simulink model "proxy_linux"  (R2017b)
settings: Solver=ode3  StartTime=0.0  StopTime=inf  FixedStep=0.01  RelTol=1e-3  EnableMultiTasking=on
model workspace (MAT data in the model file):
  SL_ROS_VariableLengthArrays_MaxSizes : struct (value not decoded)
undefined symbols (not defined in the file or in its folder): ampliFactor, ampliFactorDistal, ampliFactorMiddle, filt
libraries: robotlib x11, simulink_extras x11, simulink x8, etargetslib x4, dspnetwork x4
(part 3 of 6)

== matlab function proxy_linux/Generate SchunkCommands /Index Finger/New Version/Jacobian2 ==
  data: pose input; sensor input; measurements input; JTcomp output single; q_next output; q_pr input; J22_old input; J22_ol output
function [JTcomp, q_next, J22_ol] = fcn( pose, sensor, measurements, q_pr, J22_old)
%#codegen
% JTcomp_T = zeros(1,2);
%JTcomp = zeros(1,2);

lx = sensor(1);
qB = sensor(2);

qo1 =pose(1);
qo2 =pose(2);
qK = pose(3);
qD = pose(4);
qG = pose(5);
qN = pose(6);
c1 = pose(7);
c2 = pose(8);

%POSE ESTIMATION VALUE
LIIp = measurements(2);
LJJp = LIIp;
LLM = measurements(1);

%LIIp= measurements(1);
%LJJp = measurements(2);
%LLM = measurements(3);
%offset = measurements(4);
%xL = measurements(5);


% LIIp = 7;
% LJJp = LIIp;
% LLM = 50;
% offset = 3;
xL = 10;

f1 = LLM;
f5 = xL;
LBH = 37; 
LKB = 35;
LKH = LKB + LBH;
LCI = 16;
LGH =  86;
LHG =  LGH;
LDE = 40;
LAB =  18;   
LEF =  27;
LGF =  46;
LCD =  9;
LBC =  43;
oy  = 134.8;
ox  = 15; 
LEJ =  39;
off_fing = LIIp;  
lact = 117.77;
% LKN =  135.6320;
LNO = lact;
LDF = LDE + LEF;
LBD = LBC + LCD;


stepsize = 0.01;

%%NEWEST (Jacobian_StiffnessRenderingOptimization_Sim.mdl)
q_dif = (sensor - q_pr) / stepsize;
q_dif1 = q_dif(1);
q_dif2 = q_dif(2);


J11 = -(cos(qo1)*(LKB*cos(qK)+LBC*cos(qB-qK)-LCI*sin(qB-qK))-sin(qo1)*(LKB*sin(qK)-LBC*sin(qB-qK)-LCI*cos(qB-qK)))*((LDE+LEF)*sin(qo2)*cos(qB-qD-qG)*(LKB*sin(qK)-LBC*sin(qB-qK)-LCI*cos(qB-qK))+(LDE+LEF)*sin(qN)^2*cos(qB-qD-qG)*(cos(qo1)*sin(qo1+qo2)*(LKB*sin(qK)-LBC*sin(qB-qK))-LCI*cos(qo1)*sin(qo1+qo2)*cos(qB-qK)-sin(qo2)*(LKB*sin(qK)-LBC*sin(qB-qK)-LCI*cos(qB-qK))-sin(qo1)*cos(qo1+qo2)*(LKB*sin(qK)-LBC*sin(qB-qK)-LCI*cos(qB-qK)))-cos(qo1)*((LDE+LEF)*cos(qB-qD-qG)*(cos(qo1+qo2)*(LCD*cos(qB-qK)+LCI*sin(qB-qK)+LDE*cos(qB-qD-qK)-LEJ*sin(qB-qD-qK))-sin(qo1+qo2)*(LCI*cos(qB-qK)-LCD*sin(qB-qK)-LDE*sin(qB-qD-qK)-LEJ*cos(qB-qD-qK)))+(sin(qo1+qo2)*(LDE*sin(qB-qD-qK)+LEJ*cos(qB-qD-qK))+cos(qo1+qo2)*(LDE*cos(qB-qD-qK)-LEJ*sin(qB-qD-qK)))*(cos(qG-qK)*(LBH*cos(qK)+LHG*sin(qK)-LBC*cos(qB-qK)-LCD*cos(qB-qK)-LDE*cos(qB-qD-qK)-LEF*cos(qB-qD-qK))+sin(qG-qK)*(LHG*cos(qK)-LBH*sin(qK)-LBC*sin(qB-qK)-LCD*sin(qB-qK)-LDE*sin(qB-qD-qK)-LEF*sin(qB-qD-qK)))))/(cos(qN)*(LKB*sin(qK)+LAB*sin(qB-qK)-tan(qN)*(LKB*cos(qK)-LAB*cos(qB-qK)))*((LDE+LEF)*sin(qo1)*sin(qo2)*cos(qB-qD-qG)*(LIIp*cos(qo1)-c1*sin(qo1))*(LKB*sin(qK)-LBC*sin(qB-qK)-LCI*cos(qB-qK))-cos(qo1)*((LIIp*sin(qo1)+c1*cos(qo1))*((LDE+LEF)*sin(qo2)*cos(qB-qD-qG)*(LKB*sin(qK)-LBC*sin(qB-qK)-LCI*cos(qB-qK))-cos(qo1)*((LDE+LEF)*cos(qB-qD-qG)*(cos(qo1+qo2)*(LCD*cos(qB-qK)+LCI*sin(qB-qK)+LDE*cos(qB-qD-qK)-LEJ*sin(qB-qD-qK))-sin(qo1+qo2)*(LCI*cos(qB-qK)-LCD*sin(qB-qK)-LDE*sin(qB-qD-qK)-LEJ*cos(qB-qD-qK)))+(sin(qo1+qo2)*(LDE*sin(qB-qD-qK)+LEJ*cos(qB-qD-qK))+cos(qo1+qo2)*(LDE*cos(qB-qD-qK)-LEJ*sin(qB-qD-qK)))*(cos(qG-qK)*(LBH*cos(qK)+LHG*sin(qK)-LBC*cos(qB-qK)-LCD*cos(qB-qK)-LDE*cos(qB-qD-qK)-LEF*cos(qB-qD-qK))+sin(qG-qK)*(LHG*cos(qK)-LBH*sin(qK)-LBC*sin(qB-qK)-LCD*sin(qB-qK)-LDE*sin(qB-qD-qK)-LEF*sin(qB-qD-qK)))))-sin(qo1)*(LIIp*cos(qo1)-c1*sin(qo1))*((LDE+LEF)*sin(qo1+qo2)*cos(qB-qD-qG)*(LCI*cos(qB-qK)-LCD*sin(qB-qK)-LDE*sin(qB-qD-qK)-LEJ*cos(qB-qD-qK))-sin(qo1+qo2)*(LDE*sin(qB-qD-qK)+LEJ*cos(qB-qD-qK))*(cos(qG-qK)*(LBH*cos(qK)+LHG*sin(qK)-LBC*cos(qB-qK)-LCD*cos(qB-qK)-LDE*cos(qB-qD-qK)-LEF*cos(qB-qD-qK))+sin(qG-qK)*(LHG*cos(qK)-LBH*sin(qK)-LBC*sin(qB-qK)-LCD*sin(qB-qK)-LDE*sin(qB-qD-qK)-LEF*sin(qB-qD-qK)))-cos(qo1+qo2)*((LDE+LEF)*cos(qG-qK)*cos(qB-qD-qK)*(LCD*cos(qB-qK)+LCI*sin(qB-qK)+LDE*cos(qB-qD-qK)-LEJ*sin(qB-qD-qK))+cos(qG-qK)*(LDE*cos(qB-qD-qK)-LEJ*sin(qB-qD-qK))*(LBH*cos(qK)+LHG*sin(qK)-LBC*cos(qB-qK)-LCD*cos(qB-qK)-LDE*cos(qB-qD-qK)-LEF*cos(qB-qD-qK))+sin(qG-qK)*((LDE+LEF)*sin(qB-qD-qK)*(LCD*cos(qB-qK)+LCI*sin(qB-qK)+LDE*cos(qB-qD-qK)-LEJ*sin(qB-qD-qK))+(LDE*cos(qB-qD-qK)-LEJ*sin(qB-qD-qK))*(LHG*cos(qK)-LBH*sin(qK)-LBC*sin(qB-qK)-LCD*sin(qB-qK)-LDE*sin(qB-qD-qK)-LEF*sin(qB-qD-qK))))))));
J12 = cos(qo1)*((LDE+LEF)*sin(qo1+qo2)*cos(qB-qD-qG)*(LCI*cos(qB-qK)-LCD*sin(qB-qK)-LDE*sin(qB-qD-qK)-LEJ*cos(qB-qD-qK))*(cos(qo1)*(LKB*cos(qK)+LBC*cos(qB-qK)-LCI*sin(qB-qK))-sin(qo1)*(LKB*sin(qK)-LBC*sin(qB-qK)-LCI*cos(qB-qK)))+sin(qG-qK)*(LBC*sin(qB-qK)+LCD*sin(qB-qK)+LDE*sin(qB-qD-qK)+LEF*sin(qB-qD-qK))*(sin(qo1+qo2)*(LDE*sin(qB-qD-qK)+LEJ*cos(qB-qD-qK))+cos(qo1+qo2)*(LDE*cos(qB-qD-qK)-LEJ*sin(qB-qD-qK)))*(cos(qo1)*(LKB*cos(qK)+LBC*cos(qB-qK)-LCI*sin(qB-qK))-sin(qo1)*(LKB*sin(qK)-LBC*sin(qB-qK)-LCI*cos(qB-qK)))+cos(qG-qK)*(LBC*cos(qB-qK)+LCD*cos(qB-qK)+LDE*cos(qB-qD-qK)+LEF*cos(qB-qD-qK))*(sin(qo1+qo2)*(LDE*sin(qB-qD-qK)+LEJ*cos(qB-qD-qK))+cos(qo1+qo2)*(LDE*cos(qB-qD-qK)-LEJ*sin(qB-qD-qK)))*(cos(qo1)*(LKB*cos(qK)+LBC*cos(qB-qK)-LCI*sin(qB-qK))-sin(qo1)*(LKB*sin(qK)-LBC*sin(qB-qK)-LCI*cos(qB-qK)))-(LDE+LEF)*cos(qo1+qo2)*cos(qB-qD-qG)*(LCD*cos(qB-qK)+LCI*sin(qB-qK)+LDE*cos(qB-qD-qK)-LEJ*sin(qB-qD-qK))*(cos(qo1)*(LKB*cos(qK)+LBC*cos(qB-qK)-LCI*sin(qB-qK))-sin(qo1)*(LKB*sin(qK)-LBC*sin(qB-qK)-LCI*cos(qB-qK)))-(LBC*cos(qB-qK)-LCI*sin(qB-qK))*((LDE+LEF)*sin(qo2)*cos(qB-qD-qG)*(LKB*sin(qK)-LBC*sin(qB-qK)-LCI*cos(qB-qK))-cos(qo1)*((LDE+LEF)*cos(qB-qD-qG)*(cos(qo1+qo2)*(LCD*cos(qB-qK)+LCI*sin(qB-qK)+LDE*cos(qB-qD-qK)-LEJ*sin(qB-qD-qK))-sin(qo1+qo2)*(LCI*cos(qB-qK)-LCD*sin(qB-qK)-LDE*sin(qB-qD-qK)-LEJ*cos(qB-qD-qK)))+(sin(qo1+qo2)*(LDE*sin(qB-qD-qK)+LEJ*cos(qB-qD-qK))+cos(qo1+qo2)*(LDE*cos(qB-qD-qK)-LEJ*sin(qB-qD-qK)))*(cos(qG-qK)*(LBH*cos(qK)+LHG*sin(qK)-LBC*cos(qB-qK)-LCD*cos(qB-qK)-LDE*cos(qB-qD-qK)-LEF*cos(qB-qD-qK))+sin(qG-qK)*(LHG*cos(qK)-LBH*sin(qK)-LBC*sin(qB-qK)-LCD*sin(qB-qK)-LDE*sin(qB-qD-qK)-LEF*sin(qB-qD-qK)))))-(LBC*sin(qB-qK)+LCI*cos(qB-qK))*((LDE+LEF)*sin(qo2)*cos(qB-qD-qG)*(LKB*cos(qK)+LBC*cos(qB-qK)-LCI*sin(qB-qK))+sin(qo1)*((LDE+LEF)*sin(qo1+qo2)*cos(qB-qD-qG)*(LCI*cos(qB-qK)-LCD*sin(qB-qK)-LDE*sin(qB-qD-qK)-LEJ*cos(qB-qD-qK))-sin(qo1+qo2)*(LDE*sin(qB-qD-qK)+LEJ*cos(qB-qD-qK))*(cos(qG-qK)*(LBH*cos(qK)+LHG*sin(qK)-LBC*cos(qB-qK)-LCD*cos(qB-qK)-LDE*cos(qB-qD-qK)-LEF*cos(qB-qD-qK))+sin(qG-qK)*(LHG*cos(qK)-LBH*sin(qK)-LBC*sin(qB-qK)-LCD*sin(qB-qK)-LDE*sin(qB-qD-qK)-LEF*sin(qB-qD-qK)))-cos(qo1+qo2)*((LDE+LEF)*cos(qG-qK)*cos(qB-qD-qK)*(LCD*cos(qB-qK)+LCI*sin(qB-qK)+LDE*cos(qB-qD-qK)-LEJ*sin(qB-qD-qK))+cos(qG-qK)*(LDE*cos(qB-qD-qK)-LEJ*sin(qB-qD-qK))*(LBH*cos(qK)+LHG*sin(qK)-LBC*cos(qB-qK)-LCD*cos(qB-qK)-LDE*cos(qB-qD-qK)-LEF*cos(qB-qD-qK))+sin(qG-qK)*((LDE+LEF)*sin(qB-qD-qK)*(LCD*cos(qB-qK)+LCI*sin(qB-qK)+LDE*cos(qB-qD-qK)-LEJ*sin(qB-qD-qK))+(LDE*cos(qB-qD-qK)-LEJ*sin(qB-qD-qK))*(LHG*cos(qK)-LBH*sin(qK)-LBC*sin(qB-qK)-LCD*sin(qB-qK)-LDE*sin(qB-qD-qK)-LEF*sin(qB-qD-qK)))))))/((LDE+LEF)*sin(qo1)*sin(qo2)*cos(qB-qD-qG)*(LIIp*cos(qo1)-c1*sin(qo1))*(LKB*sin(qK)-LBC*sin(qB-qK)-LCI*cos(qB-qK))-cos(qo1)*((LIIp*sin(qo1)+c1*cos(qo1))*((LDE+LEF)*sin(qo2)*cos(qB-qD-qG)*(LKB*sin(qK)-LBC*sin(qB-qK)-LCI*cos(qB-qK))-cos(qo1)*((LDE+LEF)*cos(qB-qD-qG)*(cos(qo1+qo2)*(LCD*cos(qB-qK)+LCI*sin(qB-qK)+LDE*cos(qB-qD-qK)-LEJ*sin(qB-qD-qK))-sin(qo1+qo2)*(LCI*cos(qB-qK)-LCD*sin(qB-qK)-LDE*sin(qB-qD-qK)-LEJ*cos(qB-qD-qK)))+(sin(qo1+qo2)*(LDE*sin(qB-qD-qK)+LEJ*cos(qB-qD-qK))+cos(qo1+qo2)*(LDE*cos(qB-qD-qK)-LEJ*sin(qB-qD-qK)))*(cos(qG-qK)*(LBH*cos(qK)+LHG*sin(qK)-LBC*cos(qB-qK)-LCD*cos(qB-qK)-LDE*cos(qB-qD-qK)-LEF*cos(qB-qD-qK))+sin(qG-qK)*(LHG*cos(qK)-LBH*sin(qK)-LBC*sin(qB-qK)-LCD*sin(qB-qK)-LDE*sin(qB-qD-qK)-LEF*sin(qB-qD-qK)))))-sin(qo1)*(LIIp*cos(qo1)-c1*sin(qo1))*((LDE+LEF)*sin(qo1+qo2)*cos(qB-qD-qG)*(LCI*cos(qB-qK)-LCD*sin(qB-qK)-LDE*sin(qB-qD-qK)-LEJ*cos(qB-qD-qK))-sin(qo1+qo2)*(LDE*sin(qB-qD-qK)+LEJ*cos(qB-qD-qK))*(cos(qG-qK)*(LBH*cos(qK)+LHG*sin(qK)-LBC*cos(qB-qK)-LCD*cos(qB-qK)-LDE*cos(qB-qD-qK)-LEF*cos(qB-qD-qK))+sin(qG-qK)*(LHG*cos(qK)-LBH*sin(qK)-LBC*sin(qB-qK)-LCD*sin(qB-qK)-LDE*sin(qB-qD-qK)-LEF*sin(qB-qD-qK)))-cos(qo1+qo2)*((LDE+LEF)*cos(qG-qK)*cos(qB-qD-qK)*(LCD*cos(qB-qK)+LCI*sin(qB-qK)+LDE*cos(qB-qD-qK)-LEJ*sin(qB-qD-qK))+cos(qG-qK)*(LDE*cos(qB-qD-qK)-LEJ*sin(qB-qD-qK))*(LBH*cos(qK)+LHG*sin(qK)-LBC*cos(qB-qK)-LCD*cos(qB-qK)-LDE*cos(qB-qD-qK)-LEF*cos(qB-qD-qK))+sin(qG-qK)*((LDE+LEF)*sin(qB-qD-qK)*(LCD*cos(qB-qK)+LCI*sin(qB-qK)+LDE*cos(qB-qD-qK)-LEJ*sin(qB-qD-qK))+(LDE*cos(qB-qD-qK)-LEJ*sin(qB-qD-qK))*(LHG*cos(qK)-LBH*sin(qK)-LBC*sin(qB-qK)-LCD*sin(qB-qK)-LDE*sin(qB-qD-qK)-LEF*sin(qB-qD-qK))))))) - (cos(qo1)*(LKB*cos(qK)+LBC*cos(qB-qK)-LCI*sin(qB-qK))-sin(qo1)*(LKB*sin(qK)-LBC*sin(qB-qK)-LCI*cos(qB-qK)))*((LDE+LEF)*cos(qo1)*sin(qo1+qo2)*cos(qB-qD-qG)*(LKB*sin(qK)+LAB*sin(qB-qK)-tan(qN)*(LKB*cos(qK)-LAB*cos(qB-qK)))*(LCI*cos(qB-qK)-LCD*sin(qB-qK)-LDE*sin(qB-qD-qK)-LEJ*cos(qB-qD-qK))+cos(qo1)*sin(qG-qK)*(LKB*sin(qK)+LAB*sin(qB-qK)-tan(qN)*(LKB*cos(qK)-LAB*cos(qB-qK)))*(LBC*sin(qB-qK)+LCD*sin(qB-qK)+LDE*sin(qB-qD-qK)+LEF*sin(qB-qD-qK))*(sin(qo1+qo2)*(LDE*sin(qB-qD-qK)+LEJ*cos(qB-qD-qK))+cos(qo1+qo2)*(LDE*cos(qB-qD-qK)-LEJ*sin(qB-qD-qK)))+cos(qo1)*cos(qG-qK)*(LKB*sin(qK)+LAB*sin(qB-qK)-tan(qN)*(LKB*cos(qK)-LAB*cos(qB-qK)))*(LBC*cos(qB-qK)+LCD*cos(qB-qK)+LDE*cos(qB-qD-qK)+LEF*cos(qB-qD-qK))*(sin(qo1+qo2)*(LDE*sin(qB-qD-qK)+LEJ*cos(qB-qD-qK))+cos(qo1+qo2)*(LDE*cos(qB-qD-qK)-LEJ*sin(qB-qD-qK)))-(LDE+LEF)*sin(qo2)*cos(qB-qD-qG)*(LBC*sin(qB-qK)+LCI*cos(qB-qK))*(LKB*sin(qK)+LAB*sin(qB-qK)-tan(qN)*(LKB*cos(qK)-LAB*cos(qB-qK)))-(LDE+LEF)*cos(qo1)*cos(qo1+qo2)*cos(qB-qD-qG)*(LKB*sin(qK)+LAB*sin(qB-qK)-tan(qN)*(LKB*cos(qK)-LAB*cos(qB-qK)))*(LCD*cos(qB-qK)+LCI*sin(qB-qK)+LDE*cos(qB-qD-qK)-LEJ*sin(qB-qD-qK))-LAB*sin(qB-qK)*((LDE+LEF)*sin(qo2)*cos(qB-qD-qG)*(LKB*sin(qK)-LBC*sin(qB-qK)-LCI*cos(qB-qK))-cos(qo1)*((LDE+LEF)*cos(qB-qD-qG)*(cos(qo1+qo2)*(LCD*cos(qB-qK)+LCI*sin(qB-qK)+LDE*cos(qB-qD-qK)-LEJ*sin(qB-qD-qK))-sin(qo1+qo2)*(LCI*cos(qB-qK)-LCD*sin(qB-qK)-LDE*sin(qB-qD-qK)-LEJ*cos(qB-qD-qK)))+(sin(qo1+qo2)*(LDE*sin(qB-qD-qK)+LEJ*cos(qB-qD-qK))+cos(qo1+qo2)*(LDE*cos(qB-qD-qK)-LEJ*sin(qB-qD-qK)))*(cos(qG-qK)*(LBH*cos(qK)+LHG*sin(qK)-LBC*cos(qB-qK)-LCD*cos(qB-qK)-LDE*cos(qB-qD-qK)-LEF*cos(qB-qD-qK))+sin(qG-qK)*(LHG*cos(qK)-LBH*sin(qK)-LBC*sin(qB-qK)-LCD*sin(qB-qK)-LDE*sin(qB-qD-qK)-LEF*sin(qB-qD-qK)))))-LAB*tan(qN)*cos(qB-qK)*((LDE+LEF)*cos(qo1)*sin(qo1+qo2)*cos(qB-qD-qG)*(LKB*sin(qK)-LBC*sin(qB-qK)-LCD*sin(qB-qK)-LDE*sin(qB-qD-qK)-LEJ*cos(qB-qD-qK))-(LDE+LEF)*sin(qo1)*cos(qo1+qo2)*cos(qB-qD-qG)*(LKB*sin(qK)-LBC*sin(qB-qK)-LCI*cos(qB-qK))-cos(qo1)*sin(qo1+qo2)*(LDE*sin(qB-qD-qK)+LEJ*cos(qB-qD-qK))*(cos(qG-qK)*(LBH*cos(qK)+LHG*sin(qK)-LBC*cos(qB-qK)-LCD*cos(qB-qK)-LDE*cos(qB-qD-qK)-LEF*cos(qB-qD-qK))+sin(qG-qK)*(LHG*cos(qK)-LBH*sin(qK)-LBC*sin(qB-qK)-LCD*sin(qB-qK)-LDE*sin(qB-qD-qK)-LEF*sin(qB-qD-qK)))-cos(qo1)*cos(qo1+qo2)*((LDE+LEF)*cos(qG-qK)*cos(qB-qD-qK)*(LCD*cos(qB-qK)+LCI*sin(qB-qK)+LDE*cos(qB-qD-qK)-LEJ*sin(qB-qD-qK))+cos(qG-qK)*(LDE*cos(qB-qD-qK)-LEJ*sin(qB-qD-qK))*(LBH*cos(qK)+LHG*sin(qK)-LBC*cos(qB-qK)-LCD*cos(qB-qK)-LDE*cos(qB-qD-qK)-LEF*cos(qB-qD-qK))+sin(qG-qK)*((LDE+LEF)*sin(qB-qD-qK)*(LCD*cos(qB-qK)+LCI*sin(qB-qK)+LDE*cos(qB-qD-qK)-LEJ*sin(qB-qD-qK))+(LDE*cos(qB-qD-qK)-LEJ*sin(qB-qD-qK))*(LHG*cos(qK)-LBH*sin(qK)-LBC*sin(qB-qK)-LCD*sin(qB-qK)-LDE*sin(qB-qD-qK)-LEF*sin(qB-qD-qK))))))/((LKB*sin(qK)+LAB*sin(qB-qK)-tan(qN)*(LKB*cos(qK)-LAB*cos(qB-qK)))*((LDE+LEF)*sin(qo1)*sin(qo2)*cos(qB-qD-qG)*(LIIp*cos(qo1)-c1*sin(qo1))*(LKB*sin(qK)-LBC*sin(qB-qK)-LCI*cos(qB-qK))-cos(qo1)*((LIIp*sin(qo1)+c1*cos(qo1))*((LDE+LEF)*sin(qo2)*cos(qB-qD-qG)*(LKB*sin(qK)-LBC*sin(qB-qK)-LCI*cos(qB-qK))-cos(qo1)*((LDE+LEF)*cos(qB-qD-qG)*(cos(qo1+qo2)*(LCD*cos(qB-qK)+LCI*sin(qB-qK)+LDE*cos(qB-qD-qK)-LEJ*sin(qB-qD-qK))-sin(qo1+qo2)*(LCI*cos(qB-qK)-LCD*sin(qB-qK)-LDE*sin(qB-qD-qK)-LEJ*cos(qB-qD-qK)))+(sin(qo1+qo2)*(LDE*sin(qB-qD-qK)+LEJ*cos(qB-qD-qK))+cos(qo1+qo2)*(LDE*cos(qB-qD-qK)-LEJ*sin(qB-qD-qK)))*(cos(qG-qK)*(LBH*cos(qK)+LHG*sin(qK)-LBC*cos(qB-qK)-LCD*cos(qB-qK)-LDE*cos(qB-qD-qK)-LEF*cos(qB-qD-qK))+sin(qG-qK)*(LHG*cos(qK)-LBH*sin(qK)-LBC*sin(qB-qK)-LCD*sin(qB-qK)-LDE*sin(qB-qD-qK)-LEF*sin(qB-qD-qK)))))-sin(qo1)*(LIIp*cos(qo1)-c1*sin(qo1))*((LDE+LEF)*sin(qo1+qo2)*cos(qB-qD-qG)*(LCI*cos(qB-qK)-LCD*sin(qB-qK)-LDE*sin(qB-qD-qK)-LEJ*cos(qB-qD-qK))-sin(qo1+qo2)*(LDE*sin(qB-qD-qK)+LEJ*cos(qB-qD-qK))*(cos(qG-qK)*(LBH*cos(qK)+LHG*sin(qK)-LBC*cos(qB-qK)-LCD*cos(qB-qK)-LDE*cos(qB-qD-qK)-LEF*cos(qB-qD-qK))+sin(qG-qK)*(LHG*cos(qK)-LBH*sin(qK)-LBC*sin(qB-qK)-LCD*sin(qB-qK)-LDE*sin(qB-qD-qK)-LEF*sin(qB-qD-qK)))-cos(qo1+qo2)*((LDE+LEF)*cos(qG-qK)*cos(qB-qD-qK)*(LCD*cos(qB-qK)+LCI*sin(qB-qK)+LDE*cos(qB-qD-qK)-LEJ*sin(qB-qD-qK))+cos(qG-qK)*(LDE*cos(qB-qD-qK)-LEJ*sin(qB-qD-qK))*(LBH*cos(qK)+LHG*sin(qK)-LBC*cos(qB-qK)-LCD*cos(qB-qK)-LDE*cos(qB-qD-qK)-LEF*cos(qB-qD-qK))+sin(qG-qK)*((LDE+LEF)*sin(qB-qD-qK)*(LCD*cos(qB-qK)+LCI*sin(qB-qK)+LDE*cos(qB-qD-qK)-LEJ*sin(qB-qD-qK))+(LDE*cos(qB-qD-qK)-LEJ*sin(qB-qD-qK))*(LHG*cos(qK)-LBH*sin(qK)-LBC*sin(qB-qK)-LCD*sin(qB-qK)-LDE*sin(qB-qD-qK)-LEF*sin(qB-qD-qK))))))));
J21 = -(((LDE+LEF)*sin(qo2)*cos(qB-qD-qG)*(LKB*sin(qK)-LBC*sin(qB-qK)-LCI*cos(qB-qK))-cos(qo1)*((LDE+LEF)*cos(qB-qD-qG)*(cos(qo1+qo2)*(LCD*cos(qB-qK)+LCI*sin(qB-qK)+LDE*cos(qB-qD-qK)-LEJ*sin(qB-qD-qK))-sin(qo1+qo2)*(LCI*cos(qB-qK)-LCD*sin(qB-qK)-LDE*sin(qB-qD-qK)-LEJ*cos(qB-qD-qK)))+(sin(qo1+qo2)*(LDE*sin(qB-qD-qK)+LEJ*cos(qB-qD-qK))+cos(qo1+qo2)*(LDE*cos(qB-qD-qK)-LEJ*sin(qB-qD-qK)))*(cos(qG-qK)*(LBH*cos(qK)+LHG*sin(qK)-LBC*cos(qB-qK)-LCD*cos(qB-qK)-LDE*cos(qB-qD-qK)-LEF*cos(qB-qD-qK))+sin(qG-qK)*(LHG*cos(qK)-LBH*sin(qK)-LBC*sin(qB-qK)-LCD*sin(qB-qK)-LDE*sin(qB-qD-qK)-LEF*sin(qB-qD-qK)))))^2*(cos(qN)+sin(qN)^2*((LDE+LEF)*cos(qo1)*sin(qo1+qo2)*cos(qB-qD-qG)*(LKB*sin(qK)-LBC*sin(qB-qK)-LCD*sin(qB-qK)-LDE*sin(qB-qD-qK)-LEJ*cos(qB-qD-qK))-(LDE+LEF)*sin(qo1)*cos(qo1+qo2)*cos(qB-qD-qG)*(LKB*sin(qK)-LBC*sin(qB-qK)-LCI*cos(qB-qK))-cos(qo1)*sin(qo1+qo2)*(LDE*sin(qB-qD-qK)+LEJ*cos(qB-qD-qK))*(cos(qG-qK)*(LBH*cos(qK)+LHG*sin(qK)-LBC*cos(qB-qK)-LCD*cos(qB-qK)-LDE*cos(qB-qD-qK)-LEF*cos(qB-qD-qK))+sin(qG-qK)*(LHG*cos(qK)-LBH*sin(qK)-LBC*sin(qB-qK)-LCD*sin(qB-qK)-LDE*sin(qB-qD-qK)-LEF*sin(qB-qD-qK)))-cos(qo1)*cos(qo1+qo2)*((LDE+LEF)*cos(qG-qK)*cos(qB-qD-qK)*(LCD*cos(qB-qK)+LCI*sin(qB-qK)+LDE*cos(qB-qD-qK)-LEJ*sin(qB-qD-qK))+cos(qG-qK)*(LDE*cos(qB-qD-qK)-LEJ*sin(qB-qD-qK))*(LBH*cos(qK)+LHG*sin(qK)-LBC*cos(qB-qK)-LCD*cos(qB-qK)-LDE*cos(qB-qD-qK)-LEF*cos(qB-qD-qK))+sin(qG-qK)*((LDE+LEF)*sin(qB-qD-qK)*(LCD*cos(qB-qK)+LCI*sin(qB-qK)+LDE*cos(qB-qD-qK)-LEJ*sin(qB-qD-qK))+(LDE*cos(qB-qD-qK)-LEJ*sin(qB-qD-qK))*(LHG*cos(qK)-LBH*sin(qK)-LBC*sin(qB-qK)-LCD*sin(qB-qK)-LDE*sin(qB-qD-qK)-LEF*sin(qB-qD-qK)))))/(cos(qN)*((LDE+LEF)*sin(qo2)*cos(qB-qD-qG)*(LKB*sin(qK)-LBC*sin(qB-qK)-LCI*cos(qB-qK))-cos(qo1)*((LDE+LEF)*cos(qB-qD-qG)*(cos(qo1+qo2)*(LCD*cos(qB-qK)+LCI*sin(qB-qK)+LDE*cos(qB-qD-qK)-LEJ*sin(qB-qD-qK))-sin(qo1+qo2)*(LCI*cos(qB-qK)-LCD*sin(qB-qK)-LDE*sin(qB-qD-qK)-LEJ*cos(qB-qD-qK)))+(sin(qo1+qo2)*(LDE*sin(qB-qD-qK)+LEJ*cos(qB-qD-qK))+cos(qo1+qo2)*(LDE*cos(qB-qD-qK)-LEJ*sin(qB-qD-qK)))*(cos(qG-qK)*(LBH*cos(qK)+LHG*sin(qK)-LBC*cos(qB-qK)-LCD*cos(qB-qK)-LDE*cos(qB-qD-qK)-LEF*cos(qB-qD-qK))+sin(qG-qK)*(LHG*cos(qK)-LBH*sin(qK)-LBC*sin(qB-qK)-LCD*sin(qB-qK)-LDE*sin(qB-qD-qK)-LEF*sin(qB-qD-qK)))))))*(LIIp*sin(qo1)+c1*cos(qo1)+((LDE+LEF)*c2*cos(qB-qD-qG)*(cos(qo1)*(LKB*cos(qK)+LBC*cos(qB-qK)-LCI*sin(qB-qK))-sin(qo1)*(LKB*sin(qK)-LBC*sin(qB-qK)-LCI*cos(qB-qK)))+(LDE+LEF)*sin(qo1+qo2)*cos(qB-qD-qG)*(LIIp*cos(qo1)+sin(qo1)*(LLM-c1))*(cos(qo1)*(LKB*cos(qK)+LBC*cos(qB-qK)-LCI*sin(qB-qK))-sin(qo1)*(LKB*sin(qK)-LBC*sin(qB-qK)-LCI*cos(qB-qK)))-(LDE+LEF)*cos(qo1+qo2)*cos(qB-qD-qG)*(LIIp*sin(qo1)-cos(qo1)*(LLM-c1))*(cos(qo1)*(LKB*cos(qK)+LBC*cos(qB-qK)-LCI*sin(qB-qK))-sin(qo1)*(LKB*sin(qK)-LBC*sin(qB-qK)-LCI*cos(qB-qK)))-(LIIp*cos(qo1)-c1*sin(qo1))*((LDE+LEF)*sin(qo2)*cos(qB-qD-qG)*(LKB*cos(qK)+LBC*cos(qB-qK)-LCI*sin(qB-qK))+sin(qo1)*((LDE+LEF)*sin(qo1+qo2)*cos(qB-qD-qG)*(LCI*cos(qB-qK)-LCD*sin(qB-qK)-LDE*sin(qB-qD-qK)-LEJ*cos(qB-qD-qK))-sin(qo1+qo2)*(LDE*sin(qB-qD-qK)+LEJ*cos(qB-qD-qK))*(cos(qG-qK)*(LBH*cos(qK)+LHG*sin(qK)-LBC*cos(qB-qK)-LCD*cos(qB-qK)-LDE*cos(qB-qD-qK)-LEF*cos(qB-qD-qK))+sin(qG-qK)*(LHG*cos(qK)-LBH*sin(qK)-LBC*sin(qB-qK)-LCD*sin(qB-qK)-LDE*sin(qB-qD-qK)-LEF*sin(qB-qD-qK)))-cos(qo1+qo2)*((LDE+LEF)*cos(qG-qK)*cos(qB-qD-qK)*(LCD*cos(qB-qK)+LCI*sin(qB-qK)+LDE*cos(qB-qD-qK)-LEJ*sin(qB-qD-qK))+cos(qG-qK)*(LDE*cos(qB-qD-qK)-LEJ*sin(qB-qD-qK))*(LBH*cos(qK)+LHG*sin(qK)-LBC*cos(qB-qK)-LCD*cos(qB-qK)-LDE*cos(qB-qD-qK)-LEF*cos(qB-qD-qK))+sin(qG-qK)*((LDE+LEF)*sin(qB-qD-qK)*(LCD*cos(qB-qK)+LCI*sin(qB-qK)+LDE*cos(qB-qD-qK)-LEJ*sin(qB-qD-qK))+(LDE*cos(qB-qD-qK)-LEJ*sin(qB-qD-qK))*(LHG*cos(qK)-LBH*sin(qK)-LBC*sin(qB-qK)-LCD*sin(qB-qK)-LDE*sin(qB-qD-qK)-LEF*sin(qB-qD-qK)))))))/((LDE+LEF)*sin(qo2)*cos(qB-qD-qG)*(LKB*sin(qK)-LBC*sin(qB-qK)-LCI*cos(qB-qK))-cos(qo1)*((LDE+LEF)*cos(qB-qD-qG)*(cos(qo1+qo2)*(LCD*cos(qB-qK)+LCI*sin(qB-qK)+LDE*cos(qB-qD-qK)-LEJ*sin(qB-qD-qK))-sin(qo1+qo2)*(LCI*cos(qB-qK)-LCD*sin(qB-qK)-LDE*sin(qB-qD-qK)-LEJ*cos(qB-qD-qK)))+(sin(qo1+qo2)*(LDE*sin(qB-qD-qK)+LEJ*cos(qB-qD-qK))+cos(qo1+qo2)*(LDE*cos(qB-qD-qK)-LEJ*sin(qB-qD-qK)))*(cos(qG-qK)*(LBH*cos(qK)+LHG*sin(qK)-LBC*cos(qB-qK)-LCD*cos(qB-qK)-LDE*cos(qB-qD-qK)-LEF*cos(qB-qD-qK))+sin(qG-qK)*(LHG*cos(qK)-LBH*sin(qK)-LBC*sin(qB-qK)-LCD*sin(qB-qK)-LDE*sin(qB-qD-qK)-LEF*sin(qB-qD-qK))))))/((LDE+LEF)*c2*cos(qB-qD-qG)*(LKB*sin(qK)+LAB*sin(qB-qK)-tan(qN)*(LKB*cos(qK)-LAB*cos(qB-qK)))*((LDE+LEF)*sin(qo1)*sin(qo2)*cos(qB-qD-qG)*(LIIp*cos(qo1)-c1*sin(qo1))*(LKB*sin(qK)-LBC*sin(qB-qK)-LCI*cos(qB-qK))-cos(qo1)*((LIIp*sin(qo1)+c1*cos(qo1))*((LDE+LEF)*sin(qo2)*cos(qB-qD-qG)*(LKB*sin(qK)-LBC*sin(qB-qK)-LCI*cos(qB-qK))-cos(qo1)*((LDE+LEF)*cos(qB-qD-qG)*(cos(qo1+qo2)*(LCD*cos(qB-qK)+LCI*sin(qB-qK)+LDE*cos(qB-qD-qK)-LEJ*sin(qB-qD-qK))-sin(qo1+qo2)*(LCI*cos(qB-qK)-LCD*sin(qB-qK)-LDE*sin(qB-qD-qK)-LEJ*cos(qB-qD-qK)))+(sin(qo1+qo2)*(LDE*sin(qB-qD-qK)+LEJ*cos(qB-qD-qK))+cos(qo1+qo2)*(LDE*cos(qB-qD-qK)-LEJ*sin(qB-qD-qK)))*(cos(qG-qK)*(LBH*cos(qK)+LHG*sin(qK)-LBC*cos(qB-qK)-LCD*cos(qB-qK)-LDE*cos(qB-qD-qK)-LEF*cos(qB-qD-qK))+sin(qG-qK)*(LHG*cos(qK)-LBH*sin(qK)-LBC*sin(qB-qK)-LCD*sin(qB-qK)-LDE*sin(qB-qD-qK)-LEF*sin(qB-qD-qK)))))-sin(qo1)*(LIIp*cos(qo1)-c1*sin(qo1))*((LDE+LEF)*sin(qo1+qo2)*cos(qB-qD-qG)*(LCI*cos(qB-qK)-LCD*sin(qB-qK)-LDE*sin(qB-qD-qK)-LEJ*cos(qB-qD-qK))-sin(qo1+qo2)*(LDE*sin(qB-qD-qK)+LEJ*cos(qB-qD-qK))*(cos(qG-qK)*(LBH*cos(qK)+LHG*sin(qK)-LBC*cos(qB-qK)-LCD*cos(qB-qK)-LDE*cos(qB-qD-qK)-LEF*cos(qB-qD-qK))+sin(qG-qK)*(LHG*cos(qK)-LBH*sin(qK)-LBC*sin(qB-qK)-LCD*sin(qB-qK)-LDE*sin(qB-qD-qK)-LEF*sin(qB-qD-qK)))-cos(qo1+qo2)*((LDE+LEF)*cos(qG-qK)*cos(qB-qD-qK)*(LCD*cos(qB-qK)+LCI*sin(qB-qK)+LDE*cos(qB-qD-qK)-LEJ*sin(qB-qD-qK))+cos(qG-qK)*(LDE*cos(qB-qD-qK)-LEJ*sin(qB-qD-qK))*(LBH*cos(qK)+LHG*sin(qK)-LBC*cos(qB-qK)-LCD*cos(qB-qK)-LDE*cos(qB-qD-qK)-LEF*cos(qB-qD-qK))+sin(qG-qK)*((LDE+LEF)*sin(qB-qD-qK)*(LCD*cos(qB-qK)+LCI*sin(qB-qK)+LDE*cos(qB-qD-qK)-LEJ*sin(qB-qD-qK))+(LDE*cos(qB-qD-qK)-LEJ*sin(qB-qD-qK))*(LHG*cos(qK)-LBH*sin(qK)-LBC*sin(qB-qK)-LCD*sin(qB-qK)-LDE*sin(qB-qD-qK)-LEF*sin(qB-qD-qK)))))))));
J22_c = (-(c2*cos(qo1)+cos(qo1)*sin(qo1+qo2)*(LIIp*cos(qo1)+sin(qo1)*(LLM-c1))-sin(qo2)*(LIIp*cos(qo1)-c1*sin(qo1))-cos(qo1)*cos(qo1+qo2)*(LIIp*sin(qo1)-cos(qo1)*(LLM-c1)))*((LDE+LEF)*sin(qo1+qo2)*cos(qB-qD-qG)*(LCI*cos(qB-qK)-LCD*sin(qB-qK)-LDE*sin(qB-qD-qK)-LEJ*cos(qB-qD-qK))*(cos(qo1)*(LKB*cos(qK)+LBC*cos(qB-qK)-LCI*sin(qB-qK))-sin(qo1)*(LKB*sin(qK)-LBC*sin(qB-qK)-LCI*cos(qB-qK)))+sin(qG-qK)*(LBC*sin(qB-qK)+LCD*sin(qB-qK)+LDE*sin(qB-qD-qK)+LEF*sin(qB-qD-qK))*(sin(qo1+qo2)*(LDE*sin(qB-qD-qK)+LEJ*cos(qB-qD-qK))+cos(qo1+qo2)*(LDE*cos(qB-qD-qK)-LEJ*sin(qB-qD-qK)))*(cos(qo1)*(LKB*cos(qK)+LBC*cos(qB-qK)-LCI*sin(qB-qK))-sin(qo1)*(LKB*sin(qK)-LBC*sin(qB-qK)-LCI*cos(qB-qK)))+cos(qG-qK)*(LBC*cos(qB-qK)+LCD*cos(qB-qK)+LDE*cos(qB-qD-qK)+LEF*cos(qB-qD-qK))*(sin(qo1+qo2)*(LDE*sin(qB-qD-qK)+LEJ*cos(qB-qD-qK))+cos(qo1+qo2)*(LDE*cos(qB-qD-qK)-LEJ*sin(qB-qD-qK)))*(cos(qo1)*(LKB*cos(qK)+LBC*cos(qB-qK)-LCI*sin(qB-qK))-sin(qo1)*(LKB*sin(qK)-LBC*sin(qB-qK)-LCI*cos(qB-qK)))-(LDE+LEF)*cos(qo1+qo2)*cos(qB-qD-qG)*(LCD*cos(qB-qK)+LCI*sin(qB-qK)+LDE*cos(qB-qD-qK)-LEJ*sin(qB-qD-qK))*(cos(qo1)*(LKB*cos(qK)+LBC*cos(qB-qK)-LCI*sin(qB-qK))-sin(qo1)*(LKB*sin(qK)-LBC*sin(qB-qK)-LCI*cos(qB-qK)))-(LBC*cos(qB-qK)-LCI*sin(qB-qK))*((LDE+LEF)*sin(qo2)*cos(qB-qD-qG)*(LKB*sin(qK)-LBC*sin(qB-qK)-LCI*cos(qB-qK))-cos(qo1)*((LDE+LEF)*cos(qB-qD-qG)*(cos(qo1+qo2)*(LCD*cos(qB-qK)+LCI*sin(qB-qK)+LDE*cos(qB-qD-qK)-LEJ*sin(qB-qD-qK))-sin(qo1+qo2)*(LCI*cos(qB-qK)-LCD*sin(qB-qK)-LDE*sin(qB-qD-qK)-LEJ*cos(qB-qD-qK)))+(sin(qo1+qo2)*(LDE*sin(qB-qD-qK)+LEJ*cos(qB-qD-qK))+cos(qo1+qo2)*(LDE*cos(qB-qD-qK)-LEJ*sin(qB-qD-qK)))*(cos(qG-qK)*(LBH*cos(qK)+LHG*sin(qK)-LBC*cos(qB-qK)-LCD*cos(qB-qK)-LDE*cos(qB-qD-qK)-LEF*cos(qB-qD-qK))+sin(qG-qK)*(LHG*cos(qK)-LBH*sin(qK)-LBC*sin(qB-qK)-LCD*sin(qB-qK)-LDE*sin(qB-qD-qK)-LEF*sin(qB-qD-qK)))))-(LBC*sin(qB-qK)+LCI*cos(qB-qK))*((LDE+LEF)*sin(qo2)*cos(qB-qD-qG)*(LKB*cos(qK)+LBC*cos(qB-qK)-LCI*sin(qB-qK))+sin(qo1)*((LDE+LEF)*sin(qo1+qo2)*cos(qB-qD-qG)*(LCI*cos(qB-qK)-LCD*sin(qB-qK)-LDE*sin(qB-qD-qK)-LEJ*cos(qB-qD-qK))-sin(qo1+qo2)*(LDE*sin(qB-qD-qK)+LEJ*cos(qB-qD-qK))*(cos(qG-qK)*(LBH*cos(qK)+LHG*sin(qK)-LBC*cos(qB-qK)-LCD*cos(qB-qK)-LDE*cos(qB-qD-qK)-LEF*cos(qB-qD-qK))+sin(qG-qK)*(LHG*cos(qK)-LBH*sin(qK)-LBC*sin(qB-qK)-LCD*sin(qB-qK)-LDE*sin(qB-qD-qK)-LEF*sin(qB-qD-qK)))-cos(qo1+qo2)*((LDE+LEF)*cos(qG-qK)*cos(qB-qD-qK)*(LCD*cos(qB-qK)+LCI*sin(qB-qK)+LDE*cos(qB-qD-qK)-LEJ*sin(qB-qD-qK))+cos(qG-qK)*(LDE*cos(qB-qD-qK)-LEJ*sin(qB-qD-qK))*(LBH*cos(qK)+LHG*sin(qK)-LBC*cos(qB-qK)-LCD*cos(qB-qK)-LDE*cos(qB-qD-qK)-LEF*cos(qB-qD-qK))+sin(qG-qK)*((LDE+LEF)*sin(qB-qD-qK)*(LCD*cos(qB-qK)+LCI*sin(qB-qK)+LDE*cos(qB-qD-qK)-LEJ*sin(qB-qD-qK))+(LDE*cos(qB-qD-qK)-LEJ*sin(qB-qD-qK))*(LHG*cos(qK)-LBH*sin(qK)-LBC*sin(qB-qK)-LCD*sin(qB-qK)-LDE*sin(qB-qD-qK)-LEF*sin(qB-qD-qK)))))))/(c2*((LDE+LEF)*sin(qo1)*sin(qo2)*cos(qB-qD-qG)*(LIIp*cos(qo1)-c1*sin(qo1))*(LKB*sin(qK)-LBC*sin(qB-qK)-LCI*cos(qB-qK))-cos(qo1)*((LIIp*sin(qo1)+c1*cos(qo1))*((LDE+LEF)*sin(qo2)*cos(qB-qD-qG)*(LKB*sin(qK)-LBC*sin(qB-qK)-LCI*cos(qB-qK))-cos(qo1)*((LDE+LEF)*cos(qB-qD-qG)*(cos(qo1+qo2)*(LCD*cos(qB-qK)+LCI*sin(qB-qK)+LDE*cos(qB-qD-qK)-LEJ*sin(qB-qD-qK))-sin(qo1+qo2)*(LCI*cos(qB-qK)-LCD*sin(qB-qK)-LDE*sin(qB-qD-qK)-LEJ*cos(qB-qD-qK)))+(sin(qo1+qo2)*(LDE*sin(qB-qD-qK)+LEJ*cos(qB-qD-qK))+cos(qo1+qo2)*(LDE*cos(qB-qD-qK)-LEJ*sin(qB-qD-qK)))*(cos(qG-qK)*(LBH*cos(qK)+LHG*sin(qK)-LBC*cos(qB-qK)-LCD*cos(qB-qK)-LDE*cos(qB-qD-qK)-LEF*cos(qB-qD-qK))+sin(qG-qK)*(LHG*cos(qK)-LBH*sin(qK)-LBC*sin(qB-qK)-LCD*sin(qB-qK)-LDE*sin(qB-qD-qK)-LEF*sin(qB-qD-qK)))))-sin(qo1)*(LIIp*cos(qo1)-c1*sin(qo1))*((LDE+LEF)*sin(qo1+qo2)*cos(qB-qD-qG)*(LCI*cos(qB-qK)-LCD*sin(qB-qK)-LDE*sin(qB-qD-qK)-LEJ*cos(qB-qD-qK))-sin(qo1+qo2)*(LDE*sin(qB-qD-qK)+LEJ*cos(qB-qD-qK))*(cos(qG-qK)*(LBH*cos(qK)+LHG*sin(qK)-LBC*cos(qB-qK)-LCD*cos(qB-qK)-LDE*cos(qB-qD-qK)-LEF*cos(qB-qD-qK))+sin(qG-qK)*(LHG*cos(qK)-LBH*sin(qK)-LBC*sin(qB-qK)-LCD*sin(qB-qK)-LDE*sin(qB-qD-qK)-LEF*sin(qB-qD-qK)))-cos(qo1+qo2)*((LDE+LEF)*cos(qG-qK)*cos(qB-qD-qK)*(LCD*cos(qB-qK)+LCI*sin(qB-qK)+LDE*cos(qB-qD-qK)-LEJ*sin(qB-qD-qK))+cos(qG-qK)*(LDE*cos(qB-qD-qK)-LEJ*sin(qB-qD-qK))*(LBH*cos(qK)+LHG*sin(qK)-LBC*cos(qB-qK)-LCD*cos(qB-qK)-LDE*cos(qB-qD-qK)-LEF*cos(qB-qD-qK))+sin(qG-qK)*((LDE+LEF)*sin(qB-qD-qK)*(LCD*cos(qB-qK)+LCI*sin(qB-qK)+LDE*cos(qB-qD-qK)-LEJ*sin(qB-qD-qK))+(LDE*cos(qB-qD-qK)-LEJ*sin(qB-qD-qK))*(LHG*cos(qK)-LBH*sin(qK)-LBC*sin(qB-qK)-LCD*sin(qB-qK)-LDE*sin(qB-qD-qK)-LEF*sin(qB-qD-qK)))))))) - 2*q_dif1*abs(((LDE+LEF)*sin(qo2)*cos(qB-qD-qG)*(LKB*sin(qK)-LBC*sin(qB-qK)-LCI*cos(qB-qK))-cos(qo1)*((LDE+LEF)*cos(qB-qD-qG)*(cos(qo1+qo2)*(LCD*cos(qB-qK)+LCI*sin(qB-qK)+LDE*cos(qB-qD-qK)-LEJ*sin(qB-qD-qK))-sin(qo1+qo2)*(LCI*cos(qB-qK)-LCD*sin(qB-qK)-LDE*sin(qB-qD-qK)-LEJ*cos(qB-qD-qK)))+(sin(qo1+qo2)*(LDE*sin(qB-qD-qK)+LEJ*cos(qB-qD-qK))+cos(qo1+qo2)*(LDE*cos(qB-qD-qK)-LEJ*sin(qB-qD-qK)))*(cos(qG-qK)*(LBH*cos(qK)+LHG*sin(qK)-LBC*cos(qB-qK)-LCD*cos(qB-qK)-LDE*cos(qB-qD-qK)-LEF*cos(qB-qD-qK))+sin(qG-qK)*(LHG*cos(qK)-LBH*sin(qK)-LBC*sin(qB-qK)-LCD*sin(qB-qK)-LDE*sin(qB-qD-qK)-LEF*sin(qB-qD-qK)))))^2*(cos(qN)+sin(qN)^2*((LDE+LEF)*cos(qo1)*sin(qo1+qo2)*cos(qB-qD-qG)*(LKB*sin(qK)-LBC*sin(qB-qK)-LCD*sin(qB-qK)-LDE*sin(qB-qD-qK)-LEJ*cos(qB-qD-qK))-(LDE+LEF)*sin(qo1)*cos(qo1+qo2)*cos(qB-qD-qG)*(LKB*sin(qK)-LBC*sin(qB-qK)-LCI*cos(qB-qK))-cos(qo1)*sin(qo1+qo2)*(LDE*sin(qB-qD-qK)+LEJ*cos(qB-qD-qK))*(cos(qG-qK)*(LBH*cos(qK)+LHG*sin(qK)-LBC*cos(qB-qK)-LCD*cos(qB-qK)-LDE*cos(qB-qD-qK)-LEF*cos(qB-qD-qK))+sin(qG-qK)*(LHG*cos(qK)-LBH*sin(qK)-LBC*sin(qB-qK)-LCD*sin(qB-qK)-LDE*sin(qB-qD-qK)-LEF*sin(qB-qD-qK)))-cos(qo1)*cos(qo1+qo2)*((LDE+LEF)*cos(qG-qK)*cos(qB-qD-qK)*(LCD*cos(qB-qK)+LCI*sin(qB-qK)+LDE*cos(qB-qD-qK)-LEJ*sin(qB-qD-qK))+cos(qG-qK)*(LDE*cos(qB-qD-qK)-LEJ*sin(qB-qD-qK))*(LBH*cos(qK)+LHG*sin(qK)-LBC*cos(qB-qK)-LCD*cos(qB-qK)-LDE*cos(qB-qD-qK)-LEF*cos(qB-qD-qK))+sin(qG-qK)*((LDE+LEF)*sin(qB-qD-qK)*(LCD*cos(qB-qK)+LCI*sin(qB-qK)+LDE*cos(qB-qD-qK)-LEJ*sin(qB-qD-qK))+(LDE*cos(qB-qD-qK)-LEJ*sin(qB-qD-qK))*(LHG*cos(qK)-LBH*sin(qK)-LBC*sin(qB-qK)-LCD*sin(qB-qK)-LDE*sin(qB-qD-qK)-LEF*sin(qB-qD-qK)))))/(cos(qN)*((LDE+LEF)*sin(qo2)*cos(qB-qD-qG)*(LKB*sin(qK)-LBC*sin(qB-qK)-LCI*cos(qB-qK))-cos(qo1)*((LDE+LEF)*cos(qB-qD-qG)*(cos(qo1+qo2)*(LCD*cos(qB-qK)+LCI*sin(qB-qK)+LDE*cos(qB-qD-qK)-LEJ*sin(qB-qD-qK))-sin(qo1+qo2)*(LCI*cos(qB-qK)-LCD*sin(qB-qK)-LDE*sin(qB-qD-qK)-LEJ*cos(qB-qD-qK)))+(sin(qo1+qo2)*(LDE*sin(qB-qD-qK)+LEJ*cos(qB-qD-qK))+cos(qo1+qo2)*(LDE*cos(qB-qD-qK)-LEJ*sin(qB-qD-qK)))*(cos(qG-qK)*(LBH*cos(qK)+LHG*sin(qK)-LBC*cos(qB-qK)-LCD*cos(qB-qK)-LDE*cos(qB-qD-qK)-LEF*cos(qB-qD-qK))+sin(qG-qK)*(LHG*cos(qK)-LBH*sin(qK)-LBC*sin(qB-qK)-LCD*sin(qB-qK)-LDE*sin(qB-qD-qK)-LEF*sin(qB-qD-qK)))))))*(LIIp*sin(qo1)+c1*cos(qo1)+((LDE+LEF)*c2*cos(qB-qD-qG)*(cos(qo1)*(LKB*cos(qK)+LBC*cos(qB-qK)-LCI*sin(qB-qK))-sin(qo1)*(LKB*sin(qK)-LBC*sin(qB-qK)-LCI*cos(qB-qK)))+(LDE+LEF)*sin(qo1+qo2)*cos(qB-qD-qG)*(LIIp*cos(qo1)+sin(qo1)*(LLM-c1))*(cos(qo1)*(LKB*cos(qK)+LBC*cos(qB-qK)-LCI*sin(qB-qK))-sin(qo1)*(LKB*sin(qK)-LBC*sin(qB-qK)-LCI*cos(qB-qK)))-(LDE+LEF)*cos(qo1+qo2)*cos(qB-qD-qG)*(LIIp*sin(qo1)-cos(qo1)*(LLM-c1))*(cos(qo1)*(LKB*cos(qK)+LBC*cos(qB-qK)-LCI*sin(qB-qK))-sin(qo1)*(LKB*sin(qK)-LBC*sin(qB-qK)-LCI*cos(qB-qK)))-(LIIp*cos(qo1)-c1*sin(qo1))*((LDE+LEF)*sin(qo2)*cos(qB-qD-qG)*(LKB*cos(qK)+LBC*cos(qB-qK)-LCI*sin(qB-qK))+sin(qo1)*((LDE+LEF)*sin(qo1+qo2)*cos(qB-qD-qG)*(LCI*cos(qB-qK)-LCD*sin(qB-qK)-LDE*sin(qB-qD-qK)-LEJ*cos(qB-qD-qK))-sin(qo1+qo2)*(LDE*sin(qB-qD-qK)+LEJ*cos(qB-qD-qK))*(cos(qG-qK)*(LBH*cos(qK)+LHG*sin(qK)-LBC*cos(qB-qK)-LCD*cos(qB-qK)-LDE*cos(qB-qD-qK)-LEF*cos(qB-qD-qK))+sin(qG-qK)*(LHG*cos(qK)-LBH*sin(qK)-LBC*sin(qB-qK)-LCD*sin(qB-qK)-LDE*sin(qB-qD-qK)-LEF*sin(qB-qD-qK)))-cos(qo1+qo2)*((LDE+LEF)*cos(qG-qK)*cos(qB-qD-qK)*(LCD*cos(qB-qK)+LCI*sin(qB-qK)+LDE*cos(qB-qD-qK)-LEJ*sin(qB-qD-qK))+cos(qG-qK)*(LDE*cos(qB-qD-qK)-LEJ*sin(qB-qD-qK))*(LBH*cos(qK)+LHG*sin(qK)-LBC*cos(qB-qK)-LCD*cos(qB-qK)-LDE*cos(qB-qD-qK)-LEF*cos(qB-qD-qK))+sin(qG-qK)*((LDE+LEF)*sin(qB-qD-qK)*(LCD*cos(qB-qK)+LCI*sin(qB-qK)+LDE*cos(qB-qD-qK)-LEJ*sin(qB-qD-qK))+(LDE*cos(qB-qD-qK)-LEJ*sin(qB-qD-qK))*(LHG*cos(qK)-LBH*sin(qK)-LBC*sin(qB-qK)-LCD*sin(qB-qK)-LDE*sin(qB-qD-qK)-LEF*sin(qB-qD-qK)))))))/((LDE+LEF)*sin(qo2)*cos(qB-qD-qG)*(LKB*sin(qK)-LBC*sin(qB-qK)-LCI*cos(qB-qK))-cos(qo1)*((LDE+LEF)*cos(qB-qD-qG)*(cos(qo1+qo2)*(LCD*cos(qB-qK)+LCI*sin(qB-qK)+LDE*cos(qB-qD-qK)-LEJ*sin(qB-qD-qK))-sin(qo1+qo2)*(LCI*cos(qB-qK)-LCD*sin(qB-qK)-LDE*sin(qB-qD-qK)-LEJ*cos(qB-qD-qK)))+(sin(qo1+qo2)*(LDE*sin(qB-qD-qK)+LEJ*cos(qB-qD-qK))+cos(qo1+qo2)*(LDE*cos(qB-qD-qK)-LEJ*sin(qB-qD-qK)))*(cos(qG-qK)*(LBH*cos(qK)+LHG*sin(qK)-LBC*cos(qB-qK)-LCD*cos(qB-qK)-LDE*cos(qB-qD-qK)-LEF*cos(qB-qD-qK))+sin(qG-qK)*(LHG*cos(qK)-LBH*sin(qK)-LBC*sin(qB-qK)-LCD*sin(qB-qK)-LDE*sin(qB-qD-qK)-LEF*sin(qB-qD-qK))))))/((LDE+LEF)*c2*cos(qB-qD-qG)*(LKB*sin(qK)+LAB*sin(qB-qK)-tan(qN)*(LKB*cos(qK)-LAB*cos(qB-qK)))*((LDE+LEF)*sin(qo1)*sin(qo2)*cos(qB-qD-qG)*(LIIp*cos(qo1)-c1*sin(qo1))*(LKB*sin(qK)-LBC*sin(qB-qK)-LCI*cos(qB-qK))-cos(qo1)*((LIIp*sin(qo1)+c1*cos(qo1))*((LDE+LEF)*sin(qo2)*cos(qB-qD-qG)*(LKB*sin(qK)-LBC*sin(qB-qK)-LCI*cos(qB-qK))-cos(qo1)*((LDE+LEF)*cos(qB-qD-qG)*(cos(qo1+qo2)*(LCD*cos(qB-qK)+LCI*sin(qB-qK)+LDE*cos(qB-qD-qK)-LEJ*sin(qB-qD-qK))-sin(qo1+qo2)*(LCI*cos(qB-qK)-LCD*sin(qB-qK)-LDE*sin(qB-qD-qK)-LEJ*cos(qB-qD-qK)))+(sin(qo1+qo2)*(LDE*sin(qB-qD-qK)+LEJ*cos(qB-qD-qK))+cos(qo1+qo2)*(LDE*cos(qB-qD-qK)-LEJ*sin(qB-qD-qK)))*(cos(qG-qK)*(LBH*cos(qK)+LHG*sin(qK)-LBC*cos(qB-qK)-LCD*cos(qB-qK)-LDE*cos(qB-qD-qK)-LEF*cos(qB-qD-qK))+sin(qG-qK)*(LHG*cos(qK)-LBH*sin(qK)-LBC*sin(qB-qK)-LCD*sin(qB-qK)-LDE*sin(qB-qD-qK)-LEF*sin(qB-qD-qK)))))-sin(qo1)*(LIIp*cos(qo1)-c1*sin(qo1))*((LDE+LEF)*sin(qo1+qo2)*cos(qB-qD-qG)*(LCI*cos(qB-qK)-LCD*sin(qB-qK)-LDE*sin(qB-qD-qK)-LEJ*cos(qB-qD-qK))-sin(qo1+qo2)*(LDE*sin(qB-qD-qK)+LEJ*cos(qB-qD-qK))*(cos(qG-qK)*(LBH*cos(qK)+LHG*sin(qK)-LBC*cos(qB-qK)-LCD*cos(qB-qK)-LDE*cos(qB-qD-qK)-LEF*cos(qB-qD-qK))+sin(qG-qK)*(LHG*cos(qK)-LBH*sin(qK)-LBC*sin(qB-qK)-LCD*sin(qB-qK)-LDE*sin(qB-qD-qK)-LEF*sin(qB-qD-qK)))-cos(qo1+qo2)*((LDE+LEF)*cos(qG-qK)*cos(qB-qD-qK)*(LCD*cos(qB-qK)+LCI*sin(qB-qK)+LDE*cos(qB-qD-qK)-LEJ*sin(qB-qD-qK))+cos(qG-qK)*(LDE*cos(qB-qD-qK)-LEJ*sin(qB-qD-qK))*(LBH*cos(qK)+LHG*sin(qK)-LBC*cos(qB-qK)-LCD*cos(qB-qK)-LDE*cos(qB-qD-qK)-LEF*cos(qB-qD-qK))+sin(qG-qK)*((LDE+LEF)*sin(qB-qD-qK)*(LCD*cos(qB-qK)+LCI*sin(qB-qK)+LDE*cos(qB-qD-qK)-LEJ*sin(qB-qD-qK))+(LDE*cos(qB-qD-qK)-LEJ*sin(qB-qD-qK))*(LHG*cos(qK)-LBH*sin(qK)-LBC*sin(qB-qK)-LCD*sin(qB-qK)-LDE*sin(qB-qD-qK)-LEF*sin(qB-qD-qK)))))))))/q_dif2 - ((LDE+LEF)*sin(qo2)*cos(qB-qD-qG)*(LKB*sin(qK)-LBC*sin(qB-qK)-LCI*cos(qB-qK))-cos(qo1)*((LDE+LEF)*cos(qB-qD-qG)*(cos(qo1+qo2)*(LCD*cos(qB-qK)+LCI*sin(qB-qK)+LDE*cos(qB-qD-qK)-LEJ*sin(qB-qD-qK))-sin(qo1+qo2)*(LCI*cos(qB-qK)-LCD*sin(qB-qK)-LDE*sin(qB-qD-qK)-LEJ*cos(qB-qD-qK)))+(sin(qo1+qo2)*(LDE*sin(qB-qD-qK)+LEJ*cos(qB-qD-qK))+cos(qo1+qo2)*(LDE*cos(qB-qD-qK)-LEJ*sin(qB-qD-qK)))*(cos(qG-qK)*(LBH*cos(qK)+LHG*sin(qK)-LBC*cos(qB-qK)-LCD*cos(qB-qK)-LDE*cos(qB-qD-qK)-LEF*cos(qB-qD-qK))+sin(qG-qK)*(LHG*cos(qK)-LBH*sin(qK)-LBC*sin(qB-qK)-LCD*sin(qB-qK)-LDE*sin(qB-qD-qK)-LEF*sin(qB-qD-qK)))))^2*(LIIp*sin(qo1)+c1*cos(qo1)+((LDE+LEF)*c2*cos(qB-qD-qG)*(cos(qo1)*(LKB*cos(qK)+LBC*cos(qB-qK)-LCI*sin(qB-qK))-sin(qo1)*(LKB*sin(qK)-LBC*sin(qB-qK)-LCI*cos(qB-qK)))+(LDE+LEF)*sin(qo1+qo2)*cos(qB-qD-qG)*(LIIp*cos(qo1)+sin(qo1)*(LLM-c1))*(cos(qo1)*(LKB*cos(qK)+LBC*cos(qB-qK)-LCI*sin(qB-qK))-sin(qo1)*(LKB*sin(qK)-LBC*sin(qB-qK)-LCI*cos(qB-qK)))-(LDE+LEF)*cos(qo1+qo2)*cos(qB-qD-qG)*(LIIp*sin(qo1)-cos(qo1)*(LLM-c1))*(cos(qo1)*(LKB*cos(qK)+LBC*cos(qB-qK)-LCI*sin(qB-qK))-sin(qo1)*(LKB*sin(qK)-LBC*sin(qB-qK)-LCI*cos(qB-qK)))-(LIIp*cos(qo1)-c1*sin(qo1))*((LDE+LEF)*sin(qo2)*cos(qB-qD-qG)*(LKB*cos(qK)+LBC*cos(qB-qK)-LCI*sin(qB-qK))+sin(qo1)*((LDE+LEF)*sin(qo1+qo2)*cos(qB-qD-qG)*(LCI*cos(qB-qK)-LCD*sin(qB-qK)-LDE*sin(qB-qD-qK)-LEJ*cos(qB-qD-qK))-sin(qo1+qo2)*(LDE*sin(qB-qD-qK)+LEJ*cos(qB-qD-qK))*(cos(qG-qK)*(LBH*cos(qK)+LHG*sin(qK)-LBC*cos(qB-qK)-LCD*cos(qB-qK)-LDE*cos(qB-qD-qK)-LEF*cos(qB-qD-qK))+sin(qG-qK)*(LHG*cos(qK)-LBH*sin(qK)-LBC*sin(qB-qK)-LCD*sin(qB-qK)-LDE*sin(qB-qD-qK)-LEF*sin(qB-qD-qK)))-cos(qo1+qo2)*((LDE+LEF)*cos(qG-qK)*cos(qB-qD-qK)*(LCD*cos(qB-qK)+LCI*sin(qB-qK)+LDE*cos(qB-qD-qK)-LEJ*sin(qB-qD-qK))+cos(qG-qK)*(LDE*cos(qB-qD-qK)-LEJ*sin(qB-qD-qK))*(LBH*cos(qK)+LHG*sin(qK)-LBC*cos(qB-qK)-LCD*cos(qB-qK)-LDE*cos(qB-qD-qK)-LEF*cos(qB-qD-qK))+sin(qG-qK)*((LDE+LEF)*sin(qB-qD-qK)*(LCD*cos(qB-qK)+LCI*sin(qB-qK)+LDE*cos(qB-qD-qK)-LEJ*sin(qB-qD-qK))+(LDE*cos(qB-qD-qK)-LEJ*sin(qB-qD-qK))*(LHG*cos(qK)-LBH*sin(qK)-LBC*sin(qB-qK)-LCD*sin(qB-qK)-LDE*sin(qB-qD-qK)-LEF*sin(qB-qD-qK)))))))/((LDE+LEF)*sin(qo2)*cos(qB-qD-qG)*(LKB*sin(qK)-LBC*sin(qB-qK)-LCI*cos(qB-qK))-cos(qo1)*((LDE+LEF)*cos(qB-qD-qG)*(cos(qo1+qo2)*(LCD*cos(qB-qK)+LCI*sin(qB-qK)+LDE*cos(qB-qD-qK)-LEJ*sin(qB-qD-qK))-sin(qo1+qo2)*(LCI*cos(qB-qK)-LCD*sin(qB-qK)-LDE*sin(qB-qD-qK)-LEJ*cos(qB-qD-qK)))+(sin(qo1+qo2)*(LDE*sin(qB-qD-qK)+LEJ*cos(qB-qD-qK))+cos(qo1+qo2)*(LDE*cos(qB-qD-qK)-LEJ*sin(qB-qD-qK)))*(cos(qG-qK)*(LBH*cos(qK)+LHG*sin(qK)-LBC*cos(qB-qK)-LCD*cos(qB-qK)-LDE*cos(qB-qD-qK)-LEF*cos(qB-qD-qK))+sin(qG-qK)*(LHG*cos(qK)-LBH*sin(qK)-LBC*sin(qB-qK)-LCD*sin(qB-qK)-LDE*sin(qB-qD-qK)-LEF*sin(qB-qD-qK))))))*(LAB*sin(qB-qK)-((LDE+LEF)*cos(qo1)*sin(qo1+qo2)*cos(qB-qD-qG)*(LKB*sin(qK)+LAB*sin(qB-qK)-tan(qN)*(LKB*cos(qK)-LAB*cos(qB-qK)))*(LCI*cos(qB-qK)-LCD*sin(qB-qK)-LDE*sin(qB-qD-qK)-LEJ*cos(qB-qD-qK))+cos(qo1)*sin(qG-qK)*(LKB*sin(qK)+LAB*sin(qB-qK)-tan(qN)*(LKB*cos(qK)-LAB*cos(qB-qK)))*(LBC*sin(qB-qK)+LCD*sin(qB-qK)+LDE*sin(qB-qD-qK)+LEF*sin(qB-qD-qK))*(sin(qo1+qo2)*(LDE*sin(qB-qD-qK)+LEJ*cos(qB-qD-qK))+cos(qo1+qo2)*(LDE*cos(qB-qD-qK)-LEJ*sin(qB-qD-qK)))+cos(qo1)*cos(qG-qK)*(LKB*sin(qK)+LAB*sin(qB-qK)-tan(qN)*(LKB*cos(qK)-LAB*cos(qB-qK)))*(LBC*cos(qB-qK)+LCD*cos(qB-qK)+LDE*cos(qB-qD-qK)+LEF*cos(qB-qD-qK))*(sin(qo1+qo2)*(LDE*sin(qB-qD-qK)+LEJ*cos(qB-qD-qK))+cos(qo1+qo2)*(LDE*cos(qB-qD-qK)-LEJ*sin(qB-qD-qK)))-(LDE+LEF)*sin(qo2)*cos(qB-qD-qG)*(LBC*sin(qB-qK)+LCI*cos(qB-qK))*(LKB*sin(qK)+LAB*sin(qB-qK)-tan(qN)*(LKB*cos(qK)-LAB*cos(qB-qK)))-(LDE+LEF)*cos(qo1)*cos(qo1+qo2)*cos(qB-qD-qG)*(LKB*sin(qK)+LAB*sin(qB-qK)-tan(qN)*(LKB*cos(qK)-LAB*cos(qB-qK)))*(LCD*cos(qB-qK)+LCI*sin(qB-qK)+LDE*cos(qB-qD-qK)-LEJ*sin(qB-qD-qK))-LAB*tan(qN)*cos(qB-qK)*((LDE+LEF)*cos(qo1)*sin(qo1+qo2)*cos(qB-qD-qG)*(LKB*sin(qK)-LBC*sin(qB-qK)-LCD*sin(qB-qK)-LDE*sin(qB-qD-qK)-LEJ*cos(qB-qD-qK))-(LDE+LEF)*sin(qo1)*cos(qo1+qo2)*cos(qB-qD-qG)*(LKB*sin(qK)-LBC*sin(qB-qK)-LCI*cos(qB-qK))-cos(qo1)*sin(qo1+qo2)*(LDE*sin(qB-qD-qK)+LEJ*cos(qB-qD-qK))*(cos(qG-qK)*(LBH*cos(qK)+LHG*sin(qK)-LBC*cos(qB-qK)-LCD*cos(qB-qK)-LDE*cos(qB-qD-qK)-LEF*cos(qB-qD-qK))+sin(qG-qK)*(LHG*cos(qK)-LBH*sin(qK)-LBC*sin(qB-qK)-LCD*sin(qB-qK)-LDE*sin(qB-qD-qK)-LEF*sin(qB-qD-qK)))-cos(qo1)*cos(qo1+qo2)*((LDE+LEF)*cos(qG-qK)*cos(qB-qD-qK)*(LCD*cos(qB-qK)+LCI*sin(qB-qK)+LDE*cos(qB-qD-qK)-LEJ*sin(qB-qD-qK))+cos(qG-qK)*(LDE*cos(qB-qD-qK)-LEJ*sin(qB-qD-qK))*(LBH*cos(qK)+LHG*sin(qK)-LBC*cos(qB-qK)-LCD*cos(qB-qK)-LDE*cos(qB-qD-qK)-LEF*cos(qB-qD-qK))+sin(qG-qK)*((LDE+LEF)*sin(qB-qD-qK)*(LCD*cos(qB-qK)+LCI*sin(qB-qK)+LDE*cos(qB-qD-qK)-LEJ*sin(qB-qD-qK))+(LDE*cos(qB-qD-qK)-LEJ*sin(qB-qD-qK))*(LHG*cos(qK)-LBH*sin(qK)-LBC*sin(qB-qK)-LCD*sin(qB-qK)-LDE*sin(qB-qD-qK)-LEF*sin(qB-qD-qK))))))/((LDE+LEF)*sin(qo2)*cos(qB-qD-qG)*(LKB*sin(qK)-LBC*sin(qB-qK)-LCI*cos(qB-qK))-cos(qo1)*((LDE+LEF)*cos(qB-qD-qG)*(cos(qo1+qo2)*(LCD*cos(qB-qK)+LCI*sin(qB-qK)+LDE*cos(qB-qD-qK)-LEJ*sin(qB-qD-qK))-sin(qo1+qo2)*(LCI*cos(qB-qK)-LCD*sin(qB-qK)-LDE*sin(qB-qD-qK)-LEJ*cos(qB-qD-qK)))+(sin(qo1+qo2)*(LDE*sin(qB-qD-qK)+LEJ*cos(qB-qD-qK))+cos(qo1+qo2)*(LDE*cos(qB-qD-qK)-LEJ*sin(qB-qD-qK)))*(cos(qG-qK)*(LBH*cos(qK)+LHG*sin(qK)-LBC*cos(qB-qK)-LCD*cos(qB-qK)-LDE*cos(qB-qD-qK)-LEF*cos(qB-qD-qK))+sin(qG-qK)*(LHG*cos(qK)-LBH*sin(qK)-LBC*sin(qB-qK)-LCD*sin(qB-qK)-LDE*sin(qB-qD-qK)-LEF*sin(qB-qD-qK))))))/((LDE+LEF)*c2*cos(qB-qD-qG)*(LKB*sin(qK)+LAB*sin(qB-qK)-tan(qN)*(LKB*cos(qK)-LAB*cos(qB-qK)))*((LDE+LEF)*sin(qo1)*sin(qo2)*cos(qB-qD-qG)*(LIIp*cos(qo1)-c1*sin(qo1))*(LKB*sin(qK)-LBC*sin(qB-qK)-LCI*cos(qB-qK))-cos(qo1)*((LIIp*sin(qo1)+c1*cos(qo1))*((LDE+LEF)*sin(qo2)*cos(qB-qD-qG)*(LKB*sin(qK)-LBC*sin(qB-qK)-LCI*cos(qB-qK))-cos(qo1)*((LDE+LEF)*cos(qB-qD-qG)*(cos(qo1+qo2)*(LCD*cos(qB-qK)+LCI*sin(qB-qK)+LDE*cos(qB-qD-qK)-LEJ*sin(qB-qD-qK))-sin(qo1+qo2)*(LCI*cos(qB-qK)-LCD*sin(qB-qK)-LDE*sin(qB-qD-qK)-LEJ*cos(qB-qD-qK)))+(sin(qo1+qo2)*(LDE*sin(qB-qD-qK)+LEJ*cos(qB-qD-qK))+cos(qo1+qo2)*(LDE*cos(qB-qD-qK)-LEJ*sin(qB-qD-qK)))*(cos(qG-qK)*(LBH*cos(qK)+LHG*sin(qK)-LBC*cos(qB-qK)-LCD*cos(qB-qK)-LDE*cos(qB-qD-qK)-LEF*cos(qB-qD-qK))+sin(qG-qK)*(LHG*cos(qK)-LBH*sin(qK)-LBC*sin(qB-qK)-LCD*sin(qB-qK)-LDE*sin(qB-qD-qK)-LEF*sin(qB-qD-qK)))))-sin(qo1)*(LIIp*cos(qo1)-c1*sin(qo1))*((LDE+LEF)*sin(qo1+qo2)*cos(qB-qD-qG)*(LCI*cos(qB-qK)-LCD*sin(qB-qK)-LDE*sin(qB-qD-qK)-LEJ*cos(qB-qD-qK))-sin(qo1+qo2)*(LDE*sin(qB-qD-qK)+LEJ*cos(qB-qD-qK))*(cos(qG-qK)*(LBH*cos(qK)+LHG*sin(qK)-LBC*cos(qB-qK)-LCD*cos(qB-qK)-LDE*cos(qB-qD-qK)-LEF*cos(qB-qD-qK))+sin(qG-qK)*(LHG*cos(qK)-LBH*sin(qK)-LBC*sin(qB-qK)-LCD*sin(qB-qK)-LDE*sin(qB-qD-qK)-LEF*sin(qB-qD-qK)))-cos(qo1+qo2)*((LDE+LEF)*cos(qG-qK)*cos(qB-qD-qK)*(LCD*cos(qB-qK)+LCI*sin(qB-qK)+LDE*cos(qB-qD-qK)-LEJ*sin(qB-qD-qK))+cos(qG-qK)*(LDE*cos(qB-qD-qK)-LEJ*sin(qB-qD-qK))*(LBH*cos(qK)+LHG*sin(qK)-LBC*cos(qB-qK)-LCD*cos(qB-qK)-LDE*cos(qB-qD-qK)-LEF*cos(qB-qD-qK))+sin(qG-qK)*((LDE+LEF)*sin(qB-qD-qK)*(LCD*cos(qB-qK)+LCI*sin(qB-qK)+LDE*cos(qB-qD-qK)-LEJ*sin(qB-qD-qK))+(LDE*cos(qB-qD-qK)-LEJ*sin(qB-qD-qK))*(LHG*cos(qK)-LBH*sin(qK)-LBC*sin(qB-qK)-LCD*sin(qB-qK)-LDE*sin(qB-qD-qK)-LEF*sin(qB-qD-qK)))))))))/2;

if J22_c == 0 || isnan(J22_c) || isinf(J22_c)
    J22 = single(J22_old);
else
    J22 = single(-abs(J22_c));
end
% 
J22_ol = single(J22);



JTcomp = [J11; J12; J21; J22];


q_next = single(sensor);

== matlab function proxy_linux/Generate SchunkCommands /Index Finger/Old Version/MATLAB Function ==
  data: Jcomponents input; y output; j_f1 input; j_f2 input
function y = fcn(Jcomponents, j_f1, j_f2)
%#codegen
j_f = [j_f1;j_f2];

% JTcomp = [J11; J12; J21; J22];
JTcomp_2 = [single(Jcomponents(1)) single(Jcomponents(2)); single(Jcomponents(3)) single(Jcomponents(4))];

a_f = JTcomp_2'*j_f;
y = a_f;

== matlab function proxy_linux/ToRos/MATLAB Function - Assign ==
  data: blankMessage input; u input; msg output Bus: SL_Bus_proxy_linux_sensor_msgs_JointState; timeStamp input
function msg = assignArray(blankMessage,u,timeStamp)
%#codegen

% To set datatype of MSG output:
%  1. Create buses for this model: robotics.ros.createSimulinkBus(gcs)
%  1. Click "Edit Data" in  Toolstrip to open "Ports and Data Manager"
%  2. Select MSG and set datatype to "Bus: SL_Bus_<modelname>_<messageType>"
% See: 
% http://www.mathworks.com/help/simulink/ug/create-structures-in-matlab-function-blocks.html

% blankMessage (sensor_msgs/LaserScan) consists of 
%             Header: [1x1 Header]
%           AngleMin: 0
%           AngleMax: 0
%     AngleIncrement: 0
%      TimeIncrement: 0
%           ScanTime: 0
%           RangeMin: 0
%           RangeMax: 0
%             Ranges: [0x1 single]
%        Intensities: [0x1 single]

% Set Ranges array to have length 10, and modify indices 1, 3, 5 and 7
blankMessage.Header.Seq = timeStamp;
blankMessage.Position_SL_Info.CurrentLength = uint32(9); 
blankMessage.Position([1 2 3 4 5 6 7 8 9]) = [u(1) u(2) u(3) u(4) u(5) u(6) u(7) u(8) u(9)];
blankMessage.Velocity_SL_Info.CurrentLength = uint32(9); 
blankMessage.Velocity([1 2 3 4 5 6 7 8 9]) = zeros(1,9);
blankMessage.Effort_SL_Info.CurrentLength = uint32(9); 
blankMessage.Effort([1 2 3 4 5 6 7 8 9]) = zeros(1,9);
%blankMessage.Name.Data_SL_Info.CurrentLength = uint32(9);
%blankMessage.Name.Data([1 2 3 4 5 6 7 8 9]) = ['right_hand_Thumb_Flexion', 'right_hand_Thumb_Opposition', ...
%     'right_hand_Index_Finger_Distal','right_hand_Index_Finger_Proximal','right_hand_Middle_Finger_Distal','right_hand_Middle_Finger_Proximal',...
%     'right_hand_Ring_Finger','right_hand_Pinky','right_hand_index_spread'];

strArrayToAssign = {'right_hand_Thumb_Flexion', 'right_hand_Thumb_Opposition', ...
    'right_hand_Index_Finger_Distal','right_hand_Index_Finger_Proximal','right_hand_Middle_Finger_Distal','right_hand_Middle_Finger_Proximal',...
    'right_hand_Ring_Finger','right_hand_Pinky','right_hand_Finger_Spread'};


% Set the number of strings in the string array.
% msg (sensor_msgs/JointState) includes the following fields
%           Name : array of std_msgs/String (string array)
%   Name_SL_Info : struct with fields CurrentLength, ReceivedLength
numStringsInArray = length(strArrayToAssign);
blankMessage.Name_SL_Info.CurrentLength = uint32(numStringsInArray);

% Set the individual strings in the array
for idx=1:numStringsInArray
    str = strArrayToAssign{idx};
    strLength = length(str);
    blankMessage.Name(idx).Data(1:strLength) = uint8(str);
    blankMessage.Name(idx).Data_SL_Info.CurrentLength = uint32(strLength);
end
msg = blankMessage;
